simulink model "Simscape1"  (R2025b)
settings: Solver=FixedStepAuto  StartTime=0.0  StopTime=tend  FixedStep=TT_c  RelTol=1e-4  EnableMultiTasking=on
values from neighbouring files (symbols this model uses):
  alpha = 3.93e-3    (= 0.00393)    [Script_caricamento_dati_simscape1.m]
  alpha_PM = -0.035/100    (= -0.00035)    [Script_caricamento_dati_simscape1.m]
  Cr = In*2/4*Kc_act    (= 0.548435475)    [Script_caricamento_dati_simscape1.m]
  Crn = In*Kc_nom    (= 1.09116)    [Script_caricamento_dati_simscape1.m]
  f_AC_corr = [f_AC(1); f_AC(5:end)]    [Script_caricamento_dati_simscape1.m]
  In = 14    [Script_caricamento_dati_simscape1.m]
  isq0 = (B*wdq0/J + np*Cr0/J)/(Kc*np/J + ms*np^(2)*(Lsd-Lsq)*isd0/(2*J))    (= 0)    [Script_caricamento_dati_simscape1.m]
  J = 0.04e-3*3    (= 0.00012)    [Script_caricamento_dati_simscape1.m]
  kaisd = 1000    [Script_caricamento_dati_simscape1.m]
  kaisq = 1000    [Script_caricamento_dati_simscape1.m]
  kawr = 1000    [Script_caricamento_dati_simscape1.m]
  Kc_act = 3/2*np*PsimT    (= 0.078347925)    [Script_caricamento_dati_simscape1.m]
  kiisd = kpisd/tiisd    (= 13158.2733813)    [Script_caricamento_dati_simscape1.m]
  kiisq = kpisq/tiisq    (= 13158.2733813)    [Script_caricamento_dati_simscape1.m]
  kiPLL = 2.5e6    (= 2500000)    [Script_caricamento_dati_simscape1.m]
  kiwr = 600    [Script_caricamento_dati_simscape1.m]
  kpisd = 23.6    [Script_caricamento_dati_simscape1.m]
  kpisq = 23.6    [Script_caricamento_dati_simscape1.m]
  kpPLL = 15    [Script_caricamento_dati_simscape1.m]
  kpwr = 0.12    [Script_caricamento_dati_simscape1.m]
  lambdam_Matrix = [1 1 1; 1 1 1; 1 1 1]    [Script_caricamento_dati_simscape1.m]
  Lsd = 1.251e-3    (= 0.001251)    [Script_caricamento_dati_simscape1.m]
  Lsd_Matrix = [1 1 1; 1 1 1; 1 1 1]    [Script_caricamento_dati_simscape1.m]
  Lsq = Lsd    (= 0.001251)    [Script_caricamento_dati_simscape1.m]
  Lsq_Matrix = [1 1 1; 1 1 1; 1 1 1]    [Script_caricamento_dati_simscape1.m]
  np = 2    [Script_caricamento_dati_simscape1.m]
  np_res = 2    [Script_caricamento_dati_simscape1.m]
  Pmax = 3*Vdc/2*Imax    (= 17010)    [Script_caricamento_dati_simscape1.m]
  Psim = 26.82e-3    (= 0.02682)    [Script_caricamento_dati_simscape1.m]
  Ratio_Rs_AC = (Rs_AC_corr-Rs)/Rs    [Script_caricamento_dati_simscape1.m]
  Rs = 0.6975    [Script_caricamento_dati_simscape1.m]
  Tmax = 1.5*Crn    (= 1.63674)    [Script_caricamento_dati_simscape1.m]
  Tphase = 100    [Script_caricamento_dati_simscape1.m]
  Trif = 298.15    [Script_caricamento_dati_simscape1.m]
  Trotor = 100    [Script_caricamento_dati_simscape1.m]
  TT_c = TT_swt/100    (= 5e-07)    [Script_caricamento_dati_simscape1.m]
  TT_sc = 5e-5    (= 5e-05)    [Script_caricamento_dati_simscape1.m]
  TT_swt = 5e-5    (= 5e-05)    [Script_caricamento_dati_simscape1.m]
  Vdc = 540    [Script_caricamento_dati_simscape1.m]
  wrn = 30000    [Script_caricamento_dati_simscape1.m]
  wrr = wrn/5*1    (= 6000)    [Script_caricamento_dati_simscape1.m]
undefined symbols (not defined in the file or in its folder): denZC_id, denZC_iq, ee_sli_rtmsupport, gcbh, lambdam, numZC_id, numZC_iq
libraries: fl_lib x28, nesl_utility x22, ee_lib x14, eeTransforms x7, eeGeneralControl x6, eeDiscretePi x2, dspstat3 x1, batteryecm_lib x1, eeDqVoltageLimiter x1, eePmsmCurrentReferenceGen x1, eeVelocityController x1, eePwmGeneratorTwoLevel x1
(part 1 of 3)
settings Model: ExtModeTrigMode=oneshot  ExtModeArmWhenConnect=off  Creator=cupertinof  LastModifiedBy=Steph
settings SolverCC: AlgebraicLoopSolver=LineSearch  AutoInsertRateTranBlk=on
settings DataIOCC: SaveFormat=Array  SaveOutput=off  SaveTime=off  ReturnWorkspaceOutputs=off  SignalLoggingName=sigsOut
settings OptimizationCC: BooleanDataType=off  ConditionallyExecuteInputs=off  InitFltsAndDblsToZero=on  LifeSpan=inf
settings DebuggingCC: SaveWithParameterizedLinksMsg=none  UnderspecifiedInitializationDetection=Classic  MergeDetectMultiDrivingBlocksExec=none  SignalResolutionControl=TryResolveAllWithWarning  MultiTaskDSMMsg=warning  MultiTaskCondExecSysMsg=none  UnconnectedInputMsg=warning  UnconnectedOutputMsg=warning  UnconnectedLineMsg=warning  StateNameClashWarn=warning  SFUnexpectedBacktrackingDiag=warning  SFNoUnconditionalDefaultTransitionDiag=warning  SFExecutionAtInitializationDiag=none  ArithmeticOperatorsInVariantConditions=warning
settings HardwareCC: ProdBitPerPointer=32.0  ProdBitPerSizeT=32.0  ProdBitPerPtrDiffT=32.0  ProdLargestAtomicFloat=None  ProdIntDivRoundTo=Undefined  ProdEndianess=Unspecified  ProdWordSize=32.0  ProdHWDeviceType=32-bit Generic  TargetUnknown=on
settings ModelReferenceCC: EnableRefExpFcnMdlSchedulingChecks=on  PropagateSignalLabelsOutOfModel=off
settings SFSimCC: SimUseLocalCustomCode=off  CustomCodeUndefinedFunction=UseInterfaceOnly
settings RTWCC: RTWUseLocalCustomCode=off  GPUComputeCapability=3.5  DLArmComputeVersion=19.05
settings CodeAppCC: StateflowObjectComments=on
settings GRTTargetCC: TargetFcnLib=ansi_tfl_tmw.mat  TargetLangStandard=C89/C90 (ANSI)  CombineOutputUpdateFcns=off  GRTInterface=on
settings ConfigComp: CovMetricSettings=dw  CovSaveCumulativeToWorkspaceVar=on  CovSaveSingleToWorkspaceVar=on  CovExternalEMLEnable=off
settings SimscapeCC: SimscapeNormalizeSystem=off

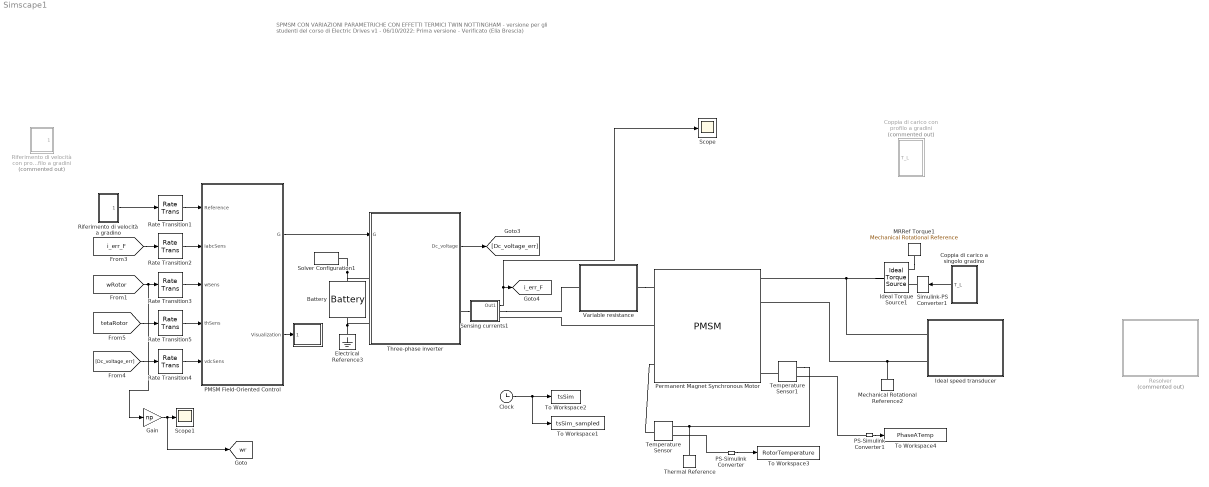
== system Simscape1 ==
  note: SPMSM CON VARIAZIONI PARAMETRICHE CON EFFETTI TERMICI TWIN NOTTINGHAM - versione per gli studenti del corso di Electric Drives
      | v1 - 06/10/2022: Prima versione - Verificato (Elia Brescia)
  " " : Subsystem
  Battery : batteryecm_lib/Battery  Vnom=Vdc V  prm_dir=1  R1_dis=2 Ohm  R1_ch=2 Ohm  R1=1e-6 Ohm  prm_AH=1  AH=14000 hr*A  V1=470 V  AH1=5000 hr*A  prm_R2=1  R2=inf Ohm  Tmeas=298.15 K  charge_measurement_port=simscape.enum.battery.enable.no  prm_dyn=1  Rp1=0.005 Ohm  tau1=30 s  Rp2=0.005 Ohm  tau2=30 s  Rp3=0.005 Ohm  tau3=30 s  Rp4=0.005 Ohm  tau4=30 s  Rp5=0.005 Ohm  tau5=30 s  prm_fade=1  N_fade=100  AH_fade=45 hr*A  R1_fade=2.02 Ohm  R1_ch_fade=2.02 Ohm  V1_fade=10.35 V  prm_age=1  prm_age_OCV=1  OCV_age=0.9  SOC_age=60  Tmeas_age=298.15 K  delta_time_age_vec=[0] d  temperature_age_vec=[273] K  OCV_scaling_age=2.2134e6  OCV_offset_age=1.632e6  temp_exp_age=0.515833569 V  t_exp_age=0.75  Vnom_T2=12 V  R1_T2=2.2 Ohm  R1_T2_dis=2.2 Ohm  R1_T2_ch=2.2 Ohm  V1_T2=11.4 V  R2_T2=2200 Ohm  Rp1_T2=0.005 Ohm  tau1_T2=30 s  Rp2_T2=0.005 Ohm  tau2_T2=30 s  Rp3_T2=0.005 Ohm  tau3_T2=30 s  Rp4_T2=0.005 Ohm  tau4_T2=30 s  Rp5_T2=0.005 Ohm  tau5_T2=30 s  Tmeas2=273.15 K  thermal_port=simscape.enum.thermaleffects.omit  thermal_mass=30000 J/K  i_specify=off  i_priority=None  i=0 A  i_nominal_specify=off  i_nominal_value=1  i_nominal_unit=A  v_specify=off  v_priority=None  v=0 V  v_nominal_specify=off  v_nominal_value=1  v_nominal_unit=V  charge_specify=on  charge_priority=High  charge=1e6 hr*A  charge_nominal_specify=off  charge_nominal_value=1  charge_nominal_unit=hr*A  num_cycles_specify=off  num_cycles_priority=High  num_cycles=0  num_cycles_nominal_specify=off  num_cycles_nominal_value=1  num_cycles_nominal_unit=1  temperature_specify=off  temperature_priority=High  temperature=298.15 K  temperature_nominal_specify=off  temperature_nominal_value=1  temperature_nominal_unit=K
  Clock : Clock
  Coppia di carico a singolo gradino : Subsystem
  Coppia di carico con profilo a gradini : Subsystem  Commented=on
  Electrical Reference3 : fl_lib/Electrical/Electrical Elements/Electrical Reference
  Gain : Gain  Gain=np
  Ideal Torque Source1 : fl_lib/Mechanical/Mechanical Sources/Ideal Torque Source
  "Ideal speed transducer " : Subsystem
  MRRef Torque1 : fl_lib/Mechanical/Rotational Elements/Mechanical Rotational Reference
  Mechanical Rotational Reference2 : fl_lib/Mechanical/Rotational Elements/Mechanical Rotational Reference
  PMSM Field-Oriented Control : Subsystem  AncestorBlock=eePmsmFieldOrientedControl/PMSM Field-Oriented Control  LoadFcn=ee_sli_rtmsupport( 'loadfcn', gcbh );  mask(PMSM Field-Oriented Control){CtrlMode=Velocity control, Vnom=Vdc, Pmax=Pmax, Tmax=Tmax, p=np, Vdc_on=10, Ts=TT_c, Tsc=TT_sc, CtrlType=PI control, Kp_w=kpwr*np*3*np*Psim/2, Ki_w=kiwr*np*3*np*Psim/2, Kv_w=1, Kaw_w=kawr, RefType=Zero d-axis control, rpmVec=[0, 3000], TqVec=[-100, 0, 100], VdcVec=[300, 350], PWMMode=SPWM: sinusoidal PWM, ModFactor=1, idMatrix=zeros(2,3,2), iqMatrix=zeros(2,3,2), psim=Psim, Ld=0.00024, Lq=0.00029, Rs=0.01, AxisAlignment=D-axis, Kp_id=kpisd, Ki_id=kiisd, Kaw_id=kaisd, Kp_iq=kpisq, Ki_iq=kiisq, Kaw_iq=kaisq, AxisPrio=D-Q equivalence, ActZC=off, ActFF=on, ParamTypeFF=Constant parameters, LdFF=Lsd, LqFF=Lsq, psimFF=Psim, idVect=[-200, 0, 200], iqVect=[-200, 0, 200], LdMatrix=0.0002 * ones(3, 3), LqMatrix=0.0002 * ones(3, 3), psimMatrix=0.04 * ones(3, 3), CPWMMode=SPWM: sinusoidal PWM, SamplingMode=Symmetric, fsw=1/TT_swt}
      mask prompts: CtrlMode "physmod:ee:library:comments:control:eePmsmFieldOrientedControl:ControlMode_MP"; Vnom "physmod:ee:library:comments:control:eePmsmFieldOrientedControl:NominalDclinkVoltageV_MP"; Pmax "physmod:ee:library:comments:control:eePmsmFieldOrientedControl:MaximumPowerW_MP"; Tmax "physmod:ee:library:comments:control:eePmsmFieldOrientedControl:MaximumTorqueNm_MP"; p "physmod:ee:library:comments:control:eePmsmFieldOrientedControl:NumberOfRotorPolePairs_MP"; Vdc_on "physmod:ee:library:comments:control:eePmsmFieldOrientedControl:InverterDclinkVoltageThresholdV_MP"; Ts "physmod:ee:library:comments:control:eePmsmFieldOrientedControl:FundamentalSampleTimes_MP"; Tsc "physmod:ee:library:comments:control:eePmsmFieldOrientedControl:ControlSampleTimes_MP"; CtrlType "physmod:ee:library:comments:control:eePmsmFieldOrientedControl:ControlType_MP"; Kp_w "physmod:ee:library:comments:control:eePmsmFieldOrientedControl:ControllerProportionalGain_MP"; Ki_w "physmod:ee:library:comments:control:eePmsmFieldOrientedControl:ControllerIntegralGain_MP"; Kv_w "physmod:ee:library:comments:control:eePmsmFieldOrientedControl:PControllerProportionalGain_MP"; Kaw_w "physmod:ee:library:comments:control:eePmsmFieldOrientedControl:IntegralAntiwindupGain_MP"; RefType "physmod:ee:library:comments:control:eePmsmFieldOrientedControl:CurrentReferences_MP"; rpmVec "physmod:ee:library:comments:control:eePmsmFieldOrientedControl:MechanicalSpeedVectorWMechanicalrpm_MP"; TqVec "physmod:ee:library:comments:control:eePmsmFieldOrientedControl:TorqueReferenceVectorTqRefNm_MP"; VdcVec "physmod:ee:library:comments:control:eePmsmFieldOrientedControl:DClinkVoltageVectorVdcV_MP"; PWMMode "physmod:ee:library:comments:control:eePmsmCurrentReferenceGen:PWMMethod_MP"; ModFactor "physmod:ee:library:comments:control:eePmsmCurrentReferenceGen:ModulationFactor_MP"; idMatrix "physmod:ee:library:comments:control:eePmsmFieldOrientedControl:DaxisCurrentReferenceMatrixIdwMechanicalTqRefVdcA_MP"; iqMatrix "physmod:ee:library:comments:control:eePmsmFieldOrientedControl:QaxisCurrentReferenceMatrixIqwMechanicalTqRefVdcA_MP"; psim "physmod:ee:library:comments:control:eePmsmFieldOrientedControl:PermanentMagnetFluxLinkageWb_MP"; Ld "physmod:ee:library:comments:control:eePmsmFieldOrientedControl:DaxisInductanceH_MP"; Lq "physmod:ee:library:comments:control:eePmsmFieldOrientedControl:QaxisInductanceH_MP"; Rs "physmod:ee:library:comments:control:eePmsmFieldOrientedControl:StatorResistanceOhm_MP"; AxisAlignment "physmod:ee:library:comments:control:eePmsmFieldOrientedControl:PhaseaAxisAlignment_MP"; Kp_id "physmod:ee:library:comments:control:eePmsmFieldOrientedControl:DaxisCurrentProportionalGain_MP"; Ki_id "physmod:ee:library:comments:control:eePmsmFieldOrientedControl:DaxisCurrentIntegralGain_MP"; Kaw_id "physmod:ee:library:comments:control:eePmsmFieldOrientedControl:DaxisCurrentAntiwindupGain_MP"; Kp_iq "physmod:ee:library:comments:control:eePmsmFieldOrientedControl:QaxisCurrentProportionalGain_MP"; Ki_iq "physmod:ee:library:comments:control:eePmsmFieldOrientedControl:QaxisCurrentIntegralGain_MP"; Kaw_iq "physmod:ee:library:comments:control:eePmsmFieldOrientedControl:QaxisCurrentAntiwindupGain_MP"; AxisPrio "physmod:ee:library:comments:control:eePmsmFieldOrientedControl:AxisPrioritization_MP"; ActZC "physmod:ee:library:comments:control:eePmsmFieldOrientedControl:EnableZeroCancellation_MP"; ActFF "physmod:ee:library:comments:control:eePmsmFieldOrientedControl:EnablePrecontrolVoltage_MP"; ParamTypeFF "physmod:ee:library:comments:control:eePmsmFieldOrientedControl:MachineParameters_MP"; LdFF "physmod:ee:library:comments:control:eePmsmFieldOrientedControl:DaxisInductanceForFeedforwardPrecontrolH_MP"; LqFF "physmod:ee:library:comments:control:eePmsmFieldOrientedControl:QaxisInductanceForFeedforwardPrecontrolH_MP"; psimFF "physmod:ee:library:comments:control:eePmsmFieldOrientedControl:PermanentMagnetFluxLinkageForFeedforwardPrecontrolWb_MP"; idVect "physmod:ee:library:comments:control:eePmsmFieldOrientedControl:DaxisCurrentVectorIdA_MP"; iqVect "physmod:ee:library:comments:control:eePmsmFieldOrientedControl:QaxisCurrentVectorIqA_MP"; LdMatrix "physmod:ee:library:comments:control:eePmsmFieldOrientedControl:LdMatrixLdidiqH_MP"; LqMatrix "physmod:ee:library:comments:control:eePmsmFieldOrientedControl:LqMatrixLqidiqH_MP"; psimMatrix "physmod:ee:library:comments:control:eePmsmFieldOrientedControl:PermanentMagnetFluxLinkageMatrixPMidiqWb_MP"; CPWMMode "physmod:ee:library:comments:control:eePmsmFieldOrientedControl:PWMMethod_MP"; SamplingMode "physmod:ee:library:comments:control:eePmsmFieldOrientedControl:SamplingMode_MP"; fsw "physmod:ee:library:comments:control:eePmsmFieldOrientedControl:SwitchingFrequencyHz_MP"
      mask help: physmod:ee:library:comments:control:eePmsmFieldOrientedControl:PMSMFieldOrientedControl_MD
      mask init:
      | if ParamTypeFF == 1
      |     idVect = [-200, 200];
      |     iqVect = [-200, 200];
      |     LdMatrix = LdFF*ones(2, 2);
      |     LqMatrix = LqFF*ones(2, 2);
      |     psimMatrix = psimFF*ones(2, 2);
      | end
      | 
      | switch CPWMMode
      |     case 'SPWM: sinusoidal PWM'
      |         set_param(gcb,'PWMMode','SPWM: sinusoidal PWM');
      |     case 'SVM: space vector modulation'
      |         set_param(gcb,'PWMMode','SVM: space vector modulation')
      | end
      settings: CopyFcn=ee_sli_rtmsupport( 'copyfcn', gcbh );  DeleteFcn=ee_sli_rtmsupport( 'deletefcn', gcbh );  ModelCloseFcn=ee_sli_rtmsupport( 'modelclosefcn', gcbh );  PostSaveFcn=ee_sli_rtmsupport( 'postsavefcn', gcbh );  PreCopyFcn=ee_sli_rtmsupport( 'precopyfcn', gcbh );  OpenFcn=ee_sli_rtmsupport( 'openfcn', gcbh );  CloseFcn=ee_sli_rtmsupport( 'closefcn', gcbh );  PreDeleteFcn=ee_sli_rtmsupport( 'predeletefcn', gcbh );
      mask Help: web(nesl_help(gcbh))
      mask TypeOptions CtrlMode: physmod:ee:library:comments:control:eePmsmFieldOrientedControl:VelocityControl_PV | physmod:ee:library:comments:control:eePmsmFieldOrientedControl:TorqueControl_PV
      mask Callback CtrlMode: ee.mask.callbackPopupPmsmFoc(gcb);
      mask TypeOptions Vnom:
      | Outer loop control/PMSM Current Reference
      | Generator/Vnom
      mask TypeOptions Pmax:
      | Outer loop control/PMSM Current Reference
      | Generator/Pmax
      mask TypeOptions Tmax:
      | Outer loop control/PMSM Current Reference
      | Generator/Tmax
      mask TypeOptions CtrlType: Outer loop control/Velocity Controller/CtrlType
      mask Callback CtrlType: ee.mask.callbackPopupPmsmFoc(gcb);
      mask TypeOptions Kp_w: Outer loop control/Velocity Controller/Kp_w
      mask TypeOptions Ki_w: Outer loop control/Velocity Controller/Ki_w
      mask TypeOptions Kv_w: Outer loop control/Velocity Controller/Kv_w
      mask TypeOptions Kaw_w: Outer loop control/Velocity Controller/Kaw_w
      mask TypeOptions RefType:
      | Outer loop control/PMSM Current Reference
      | Generator/RefType
      mask Callback RefType: ee.mask.callbackPopupPmsmFoc(gcb);
      mask TypeOptions rpmVec:
      | Outer loop control/PMSM Current Reference
      | Generator/rpmVec
      mask TypeOptions TqVec:
      | Outer loop control/PMSM Current Reference
      | Generator/TqVec
      mask TypeOptions VdcVec:
      | Outer loop control/PMSM Current Reference
      | Generator/VdcVec
      mask TypeOptions PWMMode:
      | Outer loop control/PMSM Current Reference
      | Generator/PWMMode
      mask TypeOptions ModFactor:
      | Outer loop control/PMSM Current Reference
      | Generator/ModFactor
      mask TypeOptions idMatrix:
      | Outer loop control/PMSM Current Reference
      | Generator/idMatrix
      mask TypeOptions iqMatrix:
      | Outer loop control/PMSM Current Reference
      | Generator/iqMatrix
      mask TypeOptions psim:
      | Outer loop control/PMSM Current Reference
      | Generator/psim
      mask TypeOptions Ld:
      | Outer loop control/PMSM Current Reference
      | Generator/Ld
      mask TypeOptions Lq:
      | Outer loop control/PMSM Current Reference
      | Generator/Lq
      mask TypeOptions Rs:
      | Outer loop control/PMSM Current Reference
      | Generator/Rs
      mask TypeOptions AxisAlignment: Inner loop control/Park Transform/AxisAlignment
      mask TypeOptions Kp_id:
      | Inner loop control/PMSM Current Controller
      | with Pre-Control/Kp_id
      mask TypeOptions Ki_id:
      | Inner loop control/PMSM Current Controller
      | with Pre-Control/Ki_id
      mask TypeOptions Kaw_id:
      | Inner loop control/PMSM Current Controller
      | with Pre-Control/Kaw_id
      mask TypeOptions Kp_iq:
      | Inner loop control/PMSM Current Controller
      | with Pre-Control/Kp_iq
      mask TypeOptions Ki_iq:
      | Inner loop control/PMSM Current Controller
      | with Pre-Control/Ki_iq
      mask TypeOptions Kaw_iq:
      | Inner loop control/PMSM Current Controller
      | with Pre-Control/Kaw_iq
      mask TypeOptions AxisPrio:
      | Inner loop control/PMSM Current Controller
      | with Pre-Control/AxisPrio
      mask TypeOptions ActZC:
      | Inner loop control/PMSM Current Controller
      | with Pre-Control/ActZC
      mask TypeOptions ActFF:
      | Inner loop control/PMSM Current Controller
      | with Pre-Control/ActFF
      mask Callback ActFF: ee.mask.callbackPopupPmsmFoc(gcb);
      mask TypeOptions ParamTypeFF: physmod:ee:library:comments:control:eePmsmFieldOrientedControl:ConstantParameters_PV | physmod:ee:library:comments:control:eePmsmFieldOrientedControl:LookupTableBasedParameters_PV
      mask Callback ParamTypeFF: ee.mask.callbackPopupPmsmFoc(gcb);
      mask TypeOptions idVect:
      | Inner loop control/PMSM Current Controller
      | with Pre-Control/idVect
      mask TypeOptions iqVect:
      | Inner loop control/PMSM Current Controller
      | with Pre-Control/iqVect
      mask TypeOptions LdMatrix:
      | Inner loop control/PMSM Current Controller
      | with Pre-Control/LdMatrix
      mask TypeOptions LqMatrix:
      | Inner loop control/PMSM Current Controller
      | with Pre-Control/LqMatrix
      mask TypeOptions psimMatrix:
      | Inner loop control/PMSM Current Controller
      | with Pre-Control/psimMatrix
      mask TypeOptions CPWMMode:
      | PWM/PWM Generator
      | (Three-phase, Two-level)/CPWMMode
      mask TypeOptions SamplingMode:
      | PWM/PWM Generator
      | (Three-phase, Two-level)/SamplingMode
      mask DialogControl Container4 Prompt: physmod:ee:library:comments:control:eePmsmFieldOrientedControl:tab_General
      mask DialogControl CtrlMode Prompt: Control mode
      mask DialogControl Vnom Prompt: Nominal dc-link voltage (V)
      mask DialogControl Pmax Prompt: Maximum power (W)
      mask DialogControl Tmax Prompt: Maximum torque (N*m)
      mask DialogControl p Prompt: Number of rotor pole pairs
      mask DialogControl Vdc_on Prompt: Inverter dc-link voltage threshold (V)
      mask DialogControl Ts Prompt: Fundamental sample time (s)
      mask DialogControl Tsc Prompt: Control sample time (s)
      mask DialogControl Container7 Prompt: physmod:ee:library:comments:control:eePmsmFieldOrientedControl:tab_OuterLoop
      mask DialogControl CtrlType Prompt: Control type
      mask DialogControl Kp_w Prompt: Controller proportional gain
      mask DialogControl Ki_w Prompt: Controller integral gain
      mask DialogControl Kv_w Prompt: P controller proportional gain
      mask DialogControl Kaw_w Prompt: Integral anti-windup gain
      mask DialogControl RefType Prompt: Current references
      mask DialogControl rpmVec Prompt: Mechanical speed vector, wMechanical (rpm)
      mask DialogControl TqVec Prompt: Torque reference vector, TqRef (N*m)
      mask DialogControl VdcVec Prompt: DC-link voltage vector, Vdc (V)
      mask DialogControl PWMMode Prompt: PWM method
      mask DialogControl ModFactor Prompt: Modulation factor
      mask DialogControl idMatrix Prompt: D-axis current reference matrix, id(wMechanical,TqRef,Vdc), (A)
      mask DialogControl iqMatrix Prompt: Q-axis current reference matrix, iq(wMechanical,TqRef,Vdc), (A)
      mask DialogControl psim Prompt: Permanent magnet flux linkage (Wb)
      mask DialogControl Ld Prompt: D-axis inductance (H)
      mask DialogControl Lq Prompt: Q-axis inductance (H)
      mask DialogControl Rs Prompt: Stator resistance (Ohm)
      mask DialogControl Container8 Prompt: physmod:ee:library:comments:control:eePmsmFieldOrientedControl:tab_InnerLoop
      mask DialogControl AxisAlignment Prompt: Phase-a axis alignment
      mask DialogControl Kp_id Prompt: D-axis current proportional gain
      mask DialogControl Ki_id Prompt: D-axis current integral gain
      mask DialogControl Kaw_id Prompt: D-axis current anti-windup gain
      mask DialogControl Kp_iq Prompt: Q-axis current proportional gain
      mask DialogControl Ki_iq Prompt: Q-axis current integral gain
      mask DialogControl Kaw_iq Prompt: Q-axis current anti-windup gain
      mask DialogControl AxisPrio Prompt: Axis prioritization
      mask DialogControl ActZC Prompt: Enable zero cancellation
      mask DialogControl ActFF Prompt: Enable pre-control voltage
      mask DialogControl ParamTypeFF Prompt: Machine parameters
      mask DialogControl LdFF Prompt: D-axis inductance for feed-forward pre-control (H)
      mask DialogControl LqFF Prompt: Q-axis inductance for feed-forward pre-control (H)
      mask DialogControl psimFF Prompt: Permanent magnet flux linkage for feed-forward pre-control (Wb)
      mask DialogControl idVect Prompt: D-axis current vector, id (A)
      mask DialogControl iqVect Prompt: Q-axis current vector, iq (A)
      mask DialogControl LdMatrix Prompt: Ld matrix, Ld(id,iq), (H)
      mask DialogControl LqMatrix Prompt: Lq matrix, Lq(id,iq), (H)
      mask DialogControl psimMatrix Prompt: Permanent magnet flux linkage matrix, PM(id,iq), (Wb)
      mask DialogControl Container9 Prompt: physmod:ee:library:comments:control:eePmsmFieldOrientedControl:tab_PWM
      mask DialogControl CPWMMode Prompt: PWM method
      mask DialogControl SamplingMode Prompt: Sampling mode
      mask DialogControl fsw Prompt: Switching frequency (Hz)
  PS-Simulink Converter : nesl_utility/PS-Simulink Converter  PhysicalDomain=network_engine_domain  SubClassName=ps_output  LeftPortType=input  RightPortType=output  PseudoPeriodic=off  Frequencies=[]  VectorFormat=1-D array  Unit=inherit  AffineConversion=off
  PS-Simulink Converter1 : nesl_utility/PS-Simulink Converter  PhysicalDomain=network_engine_domain  SubClassName=ps_output  LeftPortType=input  RightPortType=output  PseudoPeriodic=off  Frequencies=[]  VectorFormat=1-D array  Unit=inherit  AffineConversion=off
  Permanent Magnet Synchronous Motor : ee_lib/Electromechanical/Permanent Magnet/PMSM  port_option=ee.enum.threePhasePort.composite  winding_type=ee.enum.statorconnection.wye  machine_param=ee.enum.pmsm.parameterization.tabulated  nPolePairs=np  pmflux_param=ee.enum.pmflux.fluxlinkage  pm_flux_linkage=lambdam Wb  torque_constant=np*lambdam N*m/A  back_emf_constant=np*lambdam V/(rad/s)  stator_param=ee.enum.statorparam.LdLqL0  Ld=Lsd H  Lq=Lsq H  idVec=[-In, 0, In] A  iqVec=[-In, 0, In] A  LdMatrix=Lsd * Lsd_Matrix H  LqMatrix=Lsq * Lsq_Matrix H  PmMatrix=Psim* lambdam_Matrix Wb  ktMatrix=0.18 * ones(3, 3) N*m/A  keMatrix=0.18 * ones(3, 3) V/(rad/s)  L0=Lsd H  Ls=0.0002 H  Lm=0.00002 H  Ms=0.00002 H  Rs=Rs Ohm  zero_sequence=ee.enum.park.zerosequence.include  axes_param=ee.enum.rotorangle.daxis  loss_param=ee.enum.ironloss.none  losses_oc=[10, 10, 10] W  losses_sc=[10, 10, 10] W  f_losses=60 Hz  Isc_losses=95 A  J=J kg*m^2  lam=B N*m/(rad/s)  i_d_specify=on  i_d_priority=Low  i_d=isd0 A  i_d_nominal_specify=off  i_d_nominal_value=1  i_d_nominal_unit=A  i_q_specify=on  i_q_priority=Low  i_q=isq0 A  i_q_nominal_specify=off  i_q_nominal_value=1  i_q_nominal_unit=A  torque_specify=on  torque_priority=Low  torque=3*np*Psim*isq0/2 N*m  torque_nominal_specify=off  torque_nominal_value=1  torque_nominal_unit=N*m  angular_velocity_specify=on  angular_velocity_priority=High  angular_velocity=wr0 rad/s  angular_velocity_nominal_specify=off  angular_velocity_nominal_value=1  angular_velocity_nominal_unit=rpm  angular_position_specify=on  angular_position_priority=Low  angular_position=teta0 rad  angular_position_nominal_specify=off  angular_position_nominal_value=1  angular_position_nominal_unit=deg  alpha=alpha 1/K  alpha_flux=alpha_PM 1/K  Tmeas=Trif K  stator_thermal_mass=1e8 J/K  rotor_thermal_mass=1e8 J/K  Rm_percent_rotor=90  Rd_percent_rotor=30  temperatureA_specify=on  temperatureA_priority=Low  temperatureA=Tphase degC  temperatureA_nominal_specify=off  temperatureA_nominal_value=1  temperatureA_nominal_unit=degC  temperatureB_specify=on  temperatureB_priority=Low  temperatureB=Tphase degC  temperatureB_nominal_specify=off  temperatureB_nominal_value=1  temperatureB_nominal_unit=degC  temperatureC_specify=on  temperatureC_priority=Low  temperatureC=Tphase degC  temperatureC_nominal_specify=off  temperatureC_nominal_value=1  temperatureC_nominal_unit=degC  temperatureR_specify=on  temperatureR_priority=Low  temperatureR=Trotor degC  temperatureR_nominal_specify=off  temperatureR_nominal_value=1  temperatureR_nominal_unit=degC
      settings: LogSimulationData=on  InternalSimscapePortConfiguration="{\"Bottom\":[],\"Left\":[{\"id\":\"N\",\"label\":\"~\",\"type\":\"foundation.electrical.three_phase\"},{\"id\":\"n\",\"label\":\"n\",\"type\":\"foundation.electrical.electrical\"},{\"id\":\"HR\",\"label\":\"HR\",\"type\":\"foundation.thermal.thermal\"}],\"Right\":[{\"id\":\"R\",\"label\":\"R\",\"type\":\"foundation.mechanical.rotational.rotational\"},{\"id\":\"C\",\"label\":\"C\",\"type\":\"foundation.mechanical.rotational.rotational\"},{\"id\":\"HA\",\"label\":\"HA\",\"type\":\"foundation.thermal.thermal\"},{\"id\":\"HB\",\"label\":\"HB\",\"type\":\"foundation.thermal.thermal\"},{\"id\":\"HC\",\"label\":\"HC\",\"type\":\"foundation.thermal.thermal\"}],\"Top\":[]}"
  Rate Transition{1..5} (5 alike) : RateTransition  OutPortSampleTimeOpt=Inherit  OutPortSampleTime=TT_sc
  "Resolver " : Subsystem  Commented=on
  Riferimento di velocità a gradino : Subsystem
  Riferimento di velocità con profilo a gradini : Subsystem  Commented=on
  Scope : Scope
      settings: ActiveDisplayYMinimum=7.16843  ActiveDisplayYMaximum=8.92634  DataLoggingVariableName=ScopeData3
  Scope1 : Scope
      settings: ActiveDisplayYMinimum=-178.89975  ActiveDisplayYMaximum=1610.09776  DataLoggingVariableName=ScopeData2
  Sensing currents1 : Subsystem
      mask Display: disp('i')
  Simulink-PS Converter1 : nesl_utility/Simulink-PS Converter  PhysicalDomain=network_engine_domain  SubClassName=ps_input  LeftPortType=input  RightPortType=output  PseudoPeriodic=off  Frequencies=[]  NoiseDistribution=none  NoiseParameters=[]  Unit=N*m  AffineConversion=off  FilteringAndDerivatives=zero  SimscapeFilterOrder=1  InputFilterTimeConstant=.001  UdotUserProvided=0
  Solver Configuration1 : nesl_utility/Solver Configuration  PhysicalDomain=network_engine_domain  SubClassName=solver  LeftPortType=input  RightPortType=generic  Tones=[]  Harmonics=[]  SimulateNoise=off  Profile=off  UseLocalSampling=off  EnableSwitchedLinearOptims=on  FrequencyDomain=off  UseCCode=off  RelTol=0.001  AbsTol=1e-06  MinStep=1e-09  ToWorkspace=off  RevertToSquareIcSolve=off  NumHomotopyIterations=100  PhasorMode=off  PhasorModeNumHarmonics=1  ConsistencySolver=NEWTON_FTOL  IndexReductionMethod=DerivativeReplacement  DoDC=off  ResidualTolerance=1e-9  ConsistencyTolSource=GLOBAL  ConsistencyAbsTol=0.001  ConsistencyRelTol=0.001  ConsistencyTolFactor=0.001  UseLocalSolver=on  LocalSolverChoice=NE_BACKWARD_EULER_ADVANCER  ResolveIndetEquations=on  FunctionEvalNumThread=1  LocalSolverSampleTime=TT_c  DoFixedCost=on  MaxNonlinIter=4  MaxModeIter=2  ComputeImpulses=off  ImpulseIterations=2  LinearAlgebra=Sparse  LinearAlgebraNumThread=0  EquationFormulation=NE_TIME_EF  DelaysMemoryBudget=1024  AutomaticFiltering=on  FilteringTimeConstant=0.001  PartitionStorageMethod=AS_NEEDED  PartitionMemoryBudget=1024  PartitionMethod=FAST  MultibodyUseLocalSolver=off  MultibodyLocalSolverChoice=ODE1  MultibodyLocalSolverSampleTime=0.001
  Temperature Sensor : fl_lib/Thermal/Thermal Sensors/Temperature Sensor  temperature_measure=foundation.enum.MeasurementReference.difference
  Temperature Sensor1 : fl_lib/Thermal/Thermal Sensors/Temperature Sensor  temperature_measure=foundation.enum.MeasurementReference.difference
  Thermal Reference : fl_lib/Thermal/Thermal Elements/Thermal Reference
  Three-phase inverter : Subsystem
  To Workspace1 : ToWorkspace  VariableName=tsSim_sampled  SampleTime=TT_sc
  To Workspace2 : ToWorkspace  VariableName=tsSim  SampleTime=-1
  To Workspace3 : ToWorkspace  VariableName=RotorTemperature  SampleTime=-1
  To Workspace4 : ToWorkspace  VariableName=PhaseATemp  SampleTime=-1
  Variable resistance : Subsystem
  tag scope: i_err_F=global, wr=global
  wires:
  PMSM Field-Oriented Control/2(Visualization) -> " "/1(Variables)
  PMSM Field-Oriented Control/1(G) -> Three-phase inverter/1(G)
  Clock/1 -> To Workspace1/1, To Workspace2/1
  [Dc_voltage_err] -> Rate Transition4/1
  [tetaRotor] -> Rate Transition5/1
  Rate Transition2/1 -> PMSM Field-Oriented Control/2(iabcSens)
  Rate Transition1/1 -> PMSM Field-Oriented Control/1(Reference)
  Rate Transition3/1 -> PMSM Field-Oriented Control/3(wSens)
  Rate Transition5/1 -> PMSM Field-Oriented Control/4(thSens)
  Rate Transition4/1 -> PMSM Field-Oriented Control/5(vdcSens)
  [i_err_F] -> Rate Transition2/1
  Three-phase inverter/1(Dc_voltage) -> [Dc_voltage_err]
  Coppia di carico a singolo gradino/1(T_L) -> Simulink-PS Converter1/1
  Riferimento di velocità a gradino/1(w_ref) -> Rate Transition1/1
  PS-Simulink Converter/1 -> To Workspace3/1
  PS-Simulink Converter1/1 -> To Workspace4/1
  Sensing currents1/1(Out1) -> Scope/1, [i_err_F]
  [wRotor] -> Gain/1, Rate Transition3/1
  Gain/1 -> [wr], Scope1/1
  connections:
  Permanent Magnet Synchronous Motor/RConn2 -- "Ideal speed transducer "/LConn2 -- Mechanical Rotational Reference2/LConn1
  Ideal Torque Source1/LConn1 -- "Ideal speed transducer "/LConn1 -- Permanent Magnet Synchronous Motor/RConn1
  Three-phase inverter/RConn1 -- Sensing currents1/LConn1
  Three-phase inverter/LConn1 -- Battery/LConn1 -- Solver Configuration1/RConn1
  Electrical Reference3/LConn1 -- Three-phase inverter/LConn2 -- Battery/RConn1
  Simulink-PS Converter1/RConn1 -- Ideal Torque Source1/RConn1
  MRRef Torque1/LConn1 -- Ideal Torque Source1/RConn2
  Permanent Magnet Synchronous Motor/LConn2 -- Sensing currents1/RConn2
  Sensing currents1/RConn1 -- Variable resistance/LConn1
  Variable resistance/RConn1 -- Permanent Magnet Synchronous Motor/LConn1
  Temperature Sensor/LConn1 -- Permanent Magnet Synchronous Motor/LConn3
  Thermal Reference/LConn1 -- Temperature Sensor1/RConn1 -- Temperature Sensor/RConn1
  PS-Simulink Converter/LConn1 -- Temperature Sensor/RConn2
  PS-Simulink Converter1/LConn1 -- Temperature Sensor1/RConn2
  Temperature Sensor1/LConn1 -- Permanent Magnet Synchronous Motor/RConn5

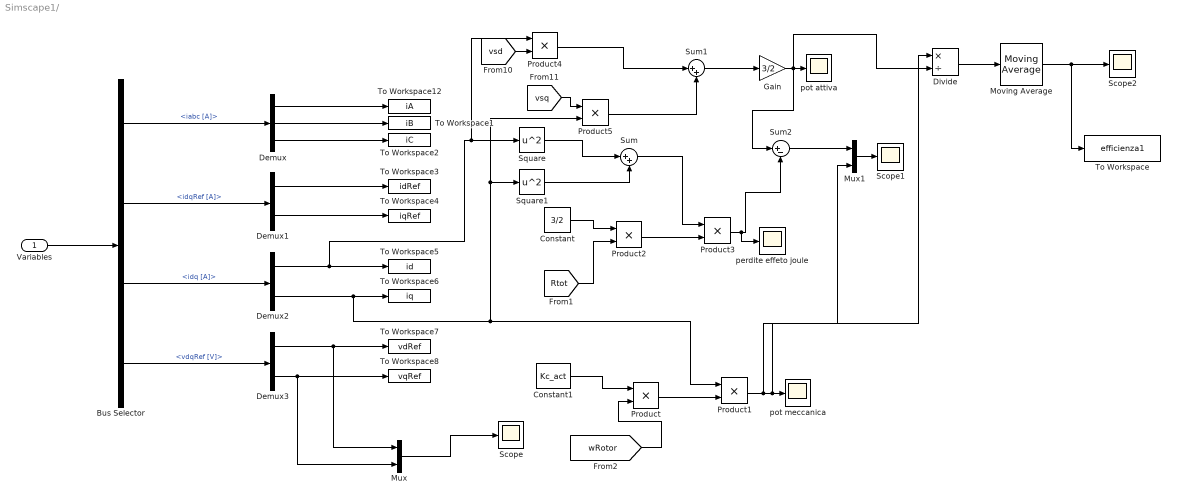
== system Simscape1/  ==
  Variables : Inport
  Bus Selector : BusSelector  OutputSignals=iabc [A],idqRef [A],idq [A],vdqRef [V]
  Constant : Constant  Value=3/2
  Constant1 : Constant  Value=Kc_act
  Demux : Demux  Outputs=3
  Demux1 : Demux  Outputs=2
  Demux2 : Demux  Outputs=2
  Demux3 : Demux  Outputs=2
  Divide : Product  Inputs=*/
  Gain : Gain  Gain=3/2
  Moving Average : dspstat3/Moving Average  Method=Sliding window  ForgettingFactorPort=off  SpecifyWindowLength=on  WindowLength=50  OverlapLength=49  AllowArbitraryInputLength=off  ForgettingFactor=0.9  SimulateUsing=Interpreted execution
  Mux : Mux  Inputs=2
  Mux1 : Mux  Inputs=2
  Product{,1..5} (6 alike) : Product
  Scope : Scope
      settings: DataLoggingVariableName=ScopeData3
  Scope1 : Scope
      settings: ActiveDisplayYMinimum=-1207.96176  ActiveDisplayYMaximum=1084.99872  DataLoggingVariableName=ScopeData5
  Scope2 : Scope
      settings: ActiveDisplayYMinimum=-0.32599  ActiveDisplayYMaximum=1.42984
  Square : Math  Operator=square
  Square1 : Math  Operator=square
  Sum : Sum  Inputs=|++
  Sum1 : Sum  Inputs=|++
  Sum2 : Sum  Inputs=|+-
  To Workspace : ToWorkspace  VariableName=efficienza1  SaveFormat=Timeseries  SampleTime=-1
  To Workspace1 : ToWorkspace  VariableName=iB  SampleTime=-1
  To Workspace12 : ToWorkspace  VariableName=iA  SampleTime=-1
  To Workspace2 : ToWorkspace  VariableName=iC  SampleTime=-1
  To Workspace3 : ToWorkspace  VariableName=idRef  SampleTime=-1
  To Workspace4 : ToWorkspace  VariableName=iqRef  SampleTime=-1
  To Workspace5 : ToWorkspace  VariableName=id  SampleTime=-1
  To Workspace6 : ToWorkspace  VariableName=iq  SampleTime=-1
  To Workspace7 : ToWorkspace  VariableName=vdRef  SampleTime=-1
  To Workspace8 : ToWorkspace  VariableName=vqRef  SampleTime=-1
  perdite effeto joule : Scope
      settings: ActiveDisplayYMinimum=-165.94479  ActiveDisplayYMaximum=1493.50314  DataLoggingVariableName=ScopeData3
  pot attiva : Scope
      settings: ActiveDisplayYMinimum=-43.8897  ActiveDisplayYMaximum=23.6103  DataLoggingVariableName=ScopeData4
  pot meccanica : Scope
      settings: ActiveDisplayYMinimum=-1230.25123  ActiveDisplayYMaximum=1435.3383  DataLoggingVariableName=ScopeData2
  wires:
  Variables/1 -> Bus Selector/1
  Bus Selector/1 -> Demux/1  "<iabc [A]>"
  Bus Selector/2 -> Demux1/1  "<idqRef [A]>"
  Bus Selector/3 -> Demux2/1  "<idq [A]>"
  Demux/1 -> To Workspace12/1
  Demux/2 -> To Workspace1/1
  Demux/3 -> To Workspace2/1
  Demux2/2 -> Product5/2, Square1/1, Product1/1, To Workspace6/1
  Demux2/1 -> Product4/1, Square/1, To Workspace5/1
  Demux1/1 -> To Workspace3/1
  Demux1/2 -> To Workspace4/1
  Bus Selector/4 -> Demux3/1  "<vdqRef [V]>"
  Demux3/2 -> Mux/2, To Workspace8/1
  Demux3/1 -> Mux/1, To Workspace7/1
  Mux/1 -> Scope/1
  Constant1/1 -> Product/1
  Product/1 -> Product1/2
  Product1/1 -> Mux1/2, Divide/1, pot meccanica/1
  [Rtot] -> Product2/2
  Constant/1 -> Product2/1
  Product2/1 -> Product3/2
  Square/1 -> Sum/1
  Square1/1 -> Sum/2
  Sum/1 -> Product3/1
  Product3/1 -> Sum2/2, perdite effeto joule/1
  [vsd] -> Product4/2
  [vsq] -> Product5/1
  Product5/1 -> Sum1/2
  Product4/1 -> Sum1/1
  Sum1/1 -> Gain/1
  Gain/1 -> Divide/2, pot attiva/1, Sum2/1
  Sum2/1 -> Mux1/1
  Mux1/1 -> Scope1/1
  [wRotor] -> Product/2
  Divide/1 -> Moving Average/1
  Moving Average/1 -> To Workspace/1, Scope2/1

== system Simscape1/Coppia di carico a singolo gradino ==
  Constant : Constant
  Gain9 : Gain  Gain=-1
  Product1 : Product  InputSameDT=on  SaturateOnIntegerOverflow=on  OutDataTypeStr=Inherit: Same as first input
  Scope : Scope
      settings: ActiveDisplayYMinimum=-0.9  ActiveDisplayYMaximum=0.1  DataLoggingVariableName=ScopeData2
  Scope1 : Scope
      settings: ActiveDisplayYMinimum=-0.025  ActiveDisplayYMaximum=0.225
  Step1 : Step  Time=0.32  After=0.4  SampleTime=0
  Step5 : Step  Time=0.12  After=0.2  SampleTime=0
  Sum : Sum  Inputs=|++
  To Workspace3 : ToWorkspace  VariableName=C_load  SampleTime=TT_sc
  T_L : Outport
  wires:
  Product1/1 -> To Workspace3/1, Scope/1, T_L/1
  Gain9/1 -> Product1/1
  Constant/1 -> Product1/2
  Step5/1 -> Sum/1
  Sum/1 -> Scope1/1, Gain9/1
  Step1/1 -> Sum/2

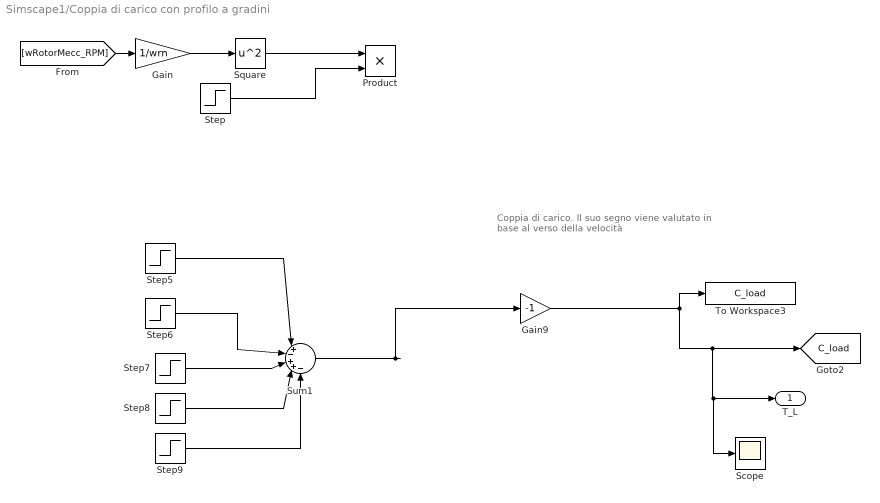
== system Simscape1/Coppia di carico con profilo a gradini ==
  note: Coppia di carico. Il suo segno viene valutato
      | in base al verso della velocità
  Gain : Gain  Gain=1/wrn
  Gain9 : Gain  Gain=-1
  Product : Product
  Scope : Scope
      settings: ActiveDisplayYMinimum=-1.8  ActiveDisplayYMaximum=0.2  DataLoggingVariableName=ScopeData2
  Square : Math  Operator=square
  Step : Step  Time=0  After=Crn  SampleTime=0
  Step5 : Step  Time=0.2  After=Cr/2  SampleTime=0
  Step6 : Step  Time=2.2  After=Cr*0.4  SampleTime=0
  Step7 : Step  Time=3.7  After=Cr*0.4  SampleTime=0
  Step8 : Step  Time=3.8  After=Cr/2  SampleTime=0
  Step9 : Step  Time=5.6  After=Cr  SampleTime=0
  Sum1 : Sum  Inputs=|+-++-
  To Workspace3 : ToWorkspace  VariableName=C_load  SampleTime=TT_sc
  T_L : Outport
  tag scope: C_load=global
  wires:
  Gain9/1 -> Scope/1, T_L/1, [C_load], To Workspace3/1
  Step9/1 -> Sum1/5
  Step6/1 -> Sum1/2
  Step8/1 -> Sum1/4
  Step5/1 -> Sum1/1
  Step7/1 -> Sum1/3
  Sum1/1 -> Gain9/1
  Square/1 -> Product/1
  Gain/1 -> Square/1
  [wRotorMecc_RPM] -> Gain/1
  Step/1 -> Product/2

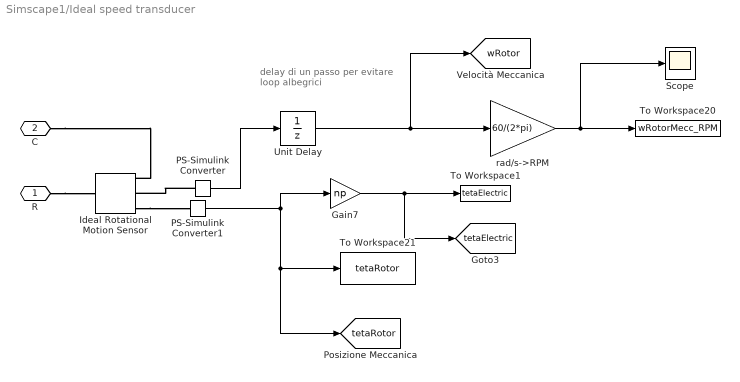
== system Simscape1/Ideal speed transducer  ==
  note: delay di un passo
      | per evitare loop albegrici
  Gain7 : Gain  Gain=np
  Ideal Rotational Motion Sensor : fl_lib/Mechanical/Mechanical Sensors/Ideal Rotational Motion Sensor  reference=foundation.enum.MeasurementReference.difference  acceleration_port=false  velocity_port=true  position_port=true  wrap_angle=simscape.enum.onoff.on  offset=0 rad
  PS-Simulink Converter : nesl_utility/PS-Simulink Converter  PhysicalDomain=network_engine_domain  SubClassName=ps_output  LeftPortType=input  RightPortType=output  PseudoPeriodic=off  Frequencies=[]  VectorFormat=1-D array  Unit=rad/s  AffineConversion=off
  PS-Simulink Converter1 : nesl_utility/PS-Simulink Converter  PhysicalDomain=network_engine_domain  SubClassName=ps_output  LeftPortType=input  RightPortType=output  PseudoPeriodic=off  Frequencies=[]  VectorFormat=1-D array  Unit=rad  AffineConversion=off
  Scope : Scope
      settings: ActiveDisplayYMinimum=-190.74206  ActiveDisplayYMaximum=1716.67858
  To Workspace1 : ToWorkspace  VariableName=tetaElectric  SampleTime=-1
  To Workspace20 : ToWorkspace  VariableName=wRotorMecc_RPM  SampleTime=TT_sc
  To Workspace21 : ToWorkspace  VariableName=tetaRotor  SampleTime=TT_sc
  Unit Delay : UnitDelay  SampleTime=-1  HasFrameUpgradeWarning=on
  rad/s->RPM : Gain  Gain=60/(2*pi)
  R : PMIOPort  Side=Left
  C : PMIOPort  Port=2  Side=Left
  tag scope: tetaElectric=global, tetaRotor=global, wRotor=global
  wires:
  Gain7/1 -> [tetaElectric], To Workspace1/1
  rad/s->RPM/1 -> Scope/1, To Workspace20/1
  PS-Simulink Converter/1 -> Unit Delay/1
  PS-Simulink Converter1/1 -> [tetaRotor], To Workspace21/1, Gain7/1
  Unit Delay/1 -> [wRotor], rad/s->RPM/1
  connections:
  R/RConn1 -- Ideal Rotational Motion Sensor/LConn1
  C/RConn1 -- Ideal Rotational Motion Sensor/RConn1
  PS-Simulink Converter/LConn1 -- Ideal Rotational Motion Sensor/RConn2
  Ideal Rotational Motion Sensor/RConn3 -- PS-Simulink Converter1/LConn1

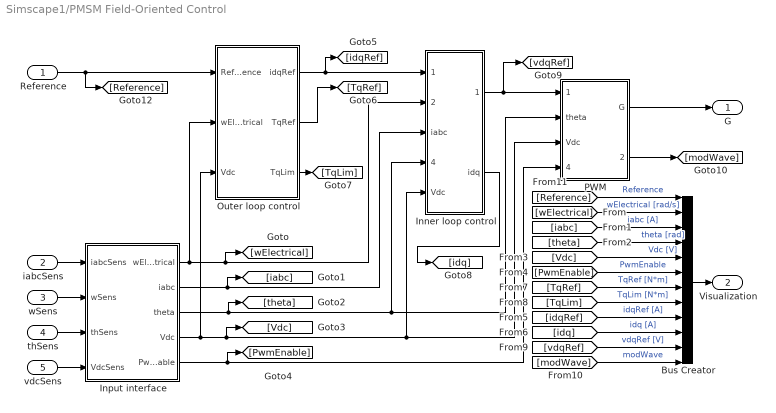
== system Simscape1/PMSM Field-Oriented Control ==
  Reference : Inport  SampleTime=Tsc
  iabcSens : Inport  Port=2  SampleTime=Tsc
  wSens : Inport  Port=3  SampleTime=Tsc
  thSens : Inport  Port=4  SampleTime=Tsc
  vdcSens : Inport  Port=5  SampleTime=Tsc
  Bus Creator : BusCreator  Inputs=12
  Inner loop control : Subsystem
  Input interface : Subsystem
  Outer loop control : Subsystem
  PWM : Subsystem
  G : Outport  VectorParamsAs1DForOutWhenUnconnected=off
  Visualization : Outport  Port=2  VectorParamsAs1DForOutWhenUnconnected=off
  wires:
  [modWave] -> Bus Creator/12  "modWave"
  [vdqRef] -> Bus Creator/11  "vdqRef [V]"
  [idq] -> Bus Creator/10  "idq [A]"
  [idqRef] -> Bus Creator/9  "idqRef [A]"
  [TqLim] -> Bus Creator/8  "TqLim [N*m]"
  [TqRef] -> Bus Creator/7  "TqRef [N*m]"
  [PwmEnable] -> Bus Creator/6  "PwmEnable"
  [Vdc] -> Bus Creator/5  "Vdc [V]"
  [theta] -> Bus Creator/4  "theta [rad]"
  [iabc] -> Bus Creator/3  "iabc [A]"
  [wElectrical] -> Bus Creator/2  "wElectrical [rad/s]"
  [Reference] -> Bus Creator/1  "Reference"
  PWM/2(ModWave) -> [modWave]
  Inner loop control/2(idq) -> [idq]
  Outer loop control/3(TqLim) -> [TqLim]
  Outer loop control/2(TqRef) -> [TqRef]
  Bus Creator/1 -> Visualization/1
  PWM/1(G) -> G/1
  Input interface/5(PwmEnable) -> PWM/4(PwmEnable), [PwmEnable]
  Inner loop control/1(vdqRef) -> PWM/1(vdqRef), [vdqRef]
  Input interface/1(wElectrical) -> Outer loop control/2(wElectrical), Inner loop control/2(wElectrical), [wElectrical]
  Input interface/4(Vdc) -> Outer loop control/3(Vdc), Inner loop control/5(Vdc), PWM/3(Vdc), [Vdc]
  Reference/1 -> Outer loop control/1(Reference), [Reference]
  vdcSens/1 -> Input interface/4(VdcSens)
  thSens/1 -> Input interface/3(thSens)
  wSens/1 -> Input interface/2(wSens)
  iabcSens/1 -> Input interface/1(iabcSens)
  Outer loop control/1(idqRef) -> Inner loop control/1(idq_ref), [idqRef]
  Input interface/3(theta) -> Inner loop control/4(theta), PWM/2(theta), [theta]
  Input interface/2(iabc) -> Inner loop control/3(iabc), [iabc]

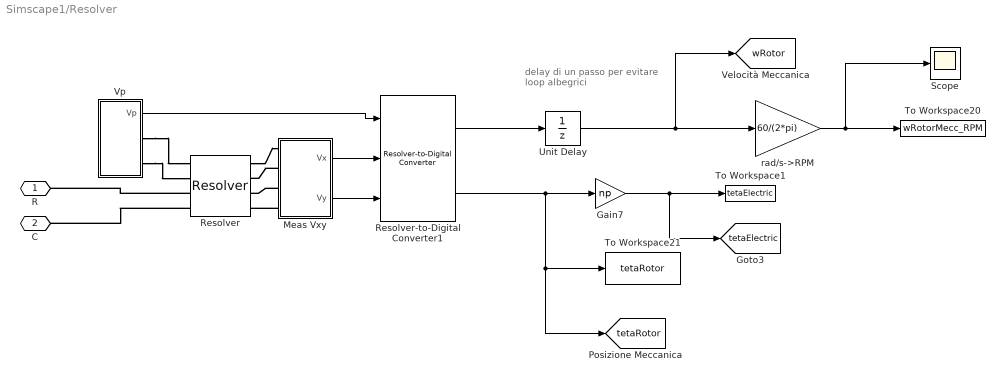
== system Simscape1/Resolver  ==
  note: delay di un passo
      | per evitare loop albegrici
  Gain7 : Gain  Gain=np
  Meas Vxy : Subsystem
  Resolver : ee_lib/Sensors & Transducers/Resolver  parameterization=2  ratio=0.5  Rr=70 Ohm  Rs=180 Ohm  Xr=100 Ohm  Xs=300 Ohm  omega=10 kHz  Lr=0.0016 H  Ls=0.0048 H  k=0.35  N=np_res  theta_specify=on  theta_priority=High  theta=teta0 rad  theta_nominal_specify=off  theta_nominal_unit=deg  theta_nominal_value=1
      settings: InternalSimscapePortConfiguration="{\"Bottom\":[],\"Left\":[{\"id\":\"p1\",\"label\":\"p1\",\"type\":\"foundation.electrical.electrical\"},{\"id\":\"p2\",\"label\":\"p2\",\"type\":\"foundation.electrical.electrical\"},{\"id\":\"R\",\"label\":\"R\",\"type\":\"foundation.mechanical.rotational.rotational\"},{\"id\":\"C\",\"label\":\"C\",\"type\":\"foundation.mechanical.rotational.rotational\"}],\"Right\":[{\"id\":\"x1\",\"label\":\"x1\",\"type\":\"foundation.electrical.electrical\"},{\"id\":\"x2\",\"label\":\"x2\",\"type\":\"foundation.electrical.electrical\"},{\"id\":\"y1\",\"label\":\"y1\",\"type\":\"foundation.electrical.electrical\"},{\"id\":\"y2\",\"label\":\"y2\",\"type\":\"foundation.electrical.electrical\"}],\"Top\":[]}"
  Resolver-to-Digital Converter1 : eeResolverToDigitalConverter/Resolver-to-Digital Converter  N=np_res  Kp=kpPLL  Ki=kiPLL  theta0=teta0  Ts=-1
  Scope : Scope
      settings: ActiveDisplayYMinimum=-358.0043  ActiveDisplayYMaximum=3222.03866
  To Workspace1 : ToWorkspace  VariableName=tetaElectric  SampleTime=-1
  To Workspace20 : ToWorkspace  VariableName=wRotorMecc_RPM  SampleTime=TT_sc
  To Workspace21 : ToWorkspace  VariableName=tetaRotor  SampleTime=TT_sc
  Unit Delay : UnitDelay  SampleTime=-1  HasFrameUpgradeWarning=on
  Vp : Subsystem
  rad/s->RPM : Gain  Gain=60/(2*pi)
  R : PMIOPort  Side=Left
  C : PMIOPort  Port=2  Side=Left
  tag scope: tetaElectric=global, tetaRotor=global, wRotor=global
  wires:
  Meas Vxy/1(Vx) -> Resolver-to-Digital Converter1/2
  Vp/1(Vp) -> Resolver-to-Digital Converter1/1
  Meas Vxy/2(Vy) -> Resolver-to-Digital Converter1/3
  Gain7/1 -> [tetaElectric], To Workspace1/1
  rad/s->RPM/1 -> Scope/1, To Workspace20/1
  Resolver-to-Digital Converter1/1 -> Unit Delay/1
  Resolver-to-Digital Converter1/2 -> Gain7/1, [tetaRotor], To Workspace21/1
  Unit Delay/1 -> [wRotor], rad/s->RPM/1
  connections:
  Vp/RConn2 -- Resolver/LConn2
  Resolver/RConn1 -- Meas Vxy/LConn1
  Resolver/LConn3 -- R/RConn1
  Meas Vxy/LConn2 -- Resolver/RConn2
  Vp/RConn1 -- Resolver/LConn1
  Meas Vxy/LConn3 -- Resolver/RConn3
  Meas Vxy/LConn4 -- Resolver/RConn4
  Resolver/LConn4 -- C/RConn1

== system Simscape1/Riferimento di velocità a gradino ==
  RPM->rad/s : Gain  Gain=(2*pi/60)
  Rate Limiter : RateLimiter  RisingSlewLimit=Tmax/J  FallingSlewLimit=-Tmax/J  SampleTimeMode=inherited
  Scope : Scope
      settings: ActiveDisplayYMinimum=21.41593  ActiveDisplayYMaximum=41.41593
  Scope1 : Scope
      settings: ActiveDisplayYMinimum=2537.72557  ActiveDisplayYMaximum=7145.26117  DataLoggingVariableName=ScopeData2
  Scope2 : Scope
      settings: ActiveDisplayYMinimum=265.75  ActiveDisplayYMaximum=748.25  DataLoggingVariableName=ScopeData2
  Step : Step  Time=0  After=314  SampleTime=0
  Step2 : Step  Time=0.2  After=386  SampleTime=0
  Sum : Sum  Inputs=|++
  To Workspace13 : ToWorkspace  VariableName=wrefRotor_RPM  SampleTime=TT_sc
  rad/s->RPM : Gain  Gain=60/(2*pi)
  w_ref : Outport
  wires:
  RPM->rad/s/1 -> w_ref/1, Scope/1
  Rate Limiter/1 -> rad/s->RPM/1
  Sum/1 -> Scope2/1, Rate Limiter/1
  rad/s->RPM/1 -> RPM->rad/s/1, Scope1/1, To Workspace13/1
  Step/1 -> Sum/1
  Step2/1 -> Sum/2

== system Simscape1/Riferimento di velocità con profilo a gradini ==
  RPM->rad/s : Gain  Gain=(2*pi/60)
  RPM->rad/s1 : Gain  Gain=(2*pi/60)
  Rate Limiter : RateLimiter  RisingSlewLimit=Tmax/J  FallingSlewLimit=-Tmax/J  SampleTimeMode=inherited
  Scope : Scope
      settings: ActiveDisplayYMinimum=-39.26991  ActiveDisplayYMaximum=353.42917
  Scope1 : Scope
      settings: ActiveDisplayYMinimum=-375  ActiveDisplayYMaximum=3375  DataLoggingVariableName=ScopeData2
  Step : Step  Time=0  After=wrr/2  SampleTime=0
  Step1 : Step  Time=2  After=wrr/2  SampleTime=0
  Step2 : Step  Time=3.5  After=0.9*wrr  SampleTime=0
  Step4 : Step  Time=5.7  After=0.1*wrr  SampleTime=0
  Sum : Sum  Inputs=|++--
  To Workspace13 : ToWorkspace  VariableName=wrefRotor_RPM  SampleTime=TT_sc
  rad/s->RPM : Gain  Gain=60/(2*pi)
  w_ref : Outport
  wires:
  RPM->rad/s/1 -> w_ref/1, Scope/1
  Rate Limiter/1 -> rad/s->RPM/1
  Step2/1 -> Sum/3
  Step1/1 -> Sum/2
  Step/1 -> Sum/1
  Step4/1 -> Sum/4
  Sum/1 -> RPM->rad/s1/1
  RPM->rad/s1/1 -> Rate Limiter/1
  rad/s->RPM/1 -> RPM->rad/s/1, Scope1/1, To Workspace13/1
